simulink model "LQG"  (R2018b)
settings: Solver=FixedStepDiscrete  StartTime=0.0  StopTime=10  FixedStep=0.02  RelTol=1e-3  EnableMultiTasking=on
values from neighbouring files (symbols this model uses):
  A = [3.3545 -4.3521 2.6058 -0.6082; 1 0 0 0; 0 1 0 0; 0 0 1 0]    [LQGm.m]    (also in Testes_planta.m = [3.11506910744011 -3.74010634305672 2.06382118501694 -0.4387)
  B = [1;0;0;0]    [LQGm.m]    (also in Testes_planta.m)
  C = [-0.0657 0.1152 0 0]    [LQGm.m]    (also in Testes_planta.m = [-0.0767099115028891 0.161398714293952 0 0])
  Nbar = Nu+K*Nx    [LQGm.m]    (also in Testes_planta.m)
undefined symbols (not defined in the file or in its folder): K, M
settings Model: Creator=user  LastModifiedBy=joaj
settings DataIOCC: LimitDataPoints=on  SaveFormat=Array
settings OptimizationCC: LifeSpan=inf
settings DebuggingCC: SFUnexpectedBacktrackingDiag=warning  SFNoUnconditionalDefaultTransitionDiag=warning  SFExecutionAtInitializationDiag=none
settings HardwareCC: ProdBitPerPointer=32  ProdBitPerSizeT=32  ProdBitPerPtrDiffT=32  ProdLargestAtomicFloat=None  ProdIntDivRoundTo=Undefined  ProdEndianess=Unspecified  ProdWordSize=32  ProdHWDeviceType=32-bit Generic
settings ModelReferenceCC: PropagateSignalLabelsOutOfModel=off
settings SFSimCC: SimUseLocalCustomCode=off
settings RTWCC: RTWUseLocalCustomCode=off
settings CodeAppCC: StateflowObjectComments=on
settings GRTTargetCC: TargetLangStandard=C89/C90 (ANSI)  GeneratePreprocessorConditionals=Disable all
settings ConfigComp: CovMetricSettings=dw  CovHtmlReporting=on  CovSaveCumulativeToWorkspaceVar=on  CovSaveSingleToWorkspaceVar=on  CovExternalEMLEnable=off

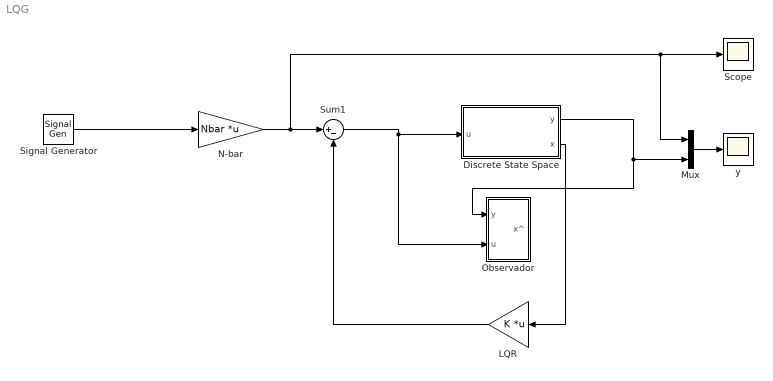
== system LQG ==
  "Discrete State Space " : Subsystem
  LQR : Gain  Gain=K  Multiplication=Matrix(K*u)
  Mux : Mux  Inputs=2
  N-bar : Gain  Gain=Nbar  Multiplication=Matrix(K*u)
  Observador : Subsystem
  Scope : Scope
  Signal Generator : SignalGenerator  WaveForm=square  Amplitude=90  Frequency=0.4
  Sum1 : Sum  Inputs=|+-
  y : Scope
  wires:
  LQR/1 -> Sum1/2
  "Discrete State Space "/1(y) -> Mux/2, Observador/1(y)
  Sum1/1 -> Observador/2(u), "Discrete State Space "/1(u)
  N-bar/1 -> Mux/1, Scope/1, Sum1/1
  "Discrete State Space "/2(x) -> LQR/1
  Signal Generator/1 -> N-bar/1
  Mux/1 -> y/1

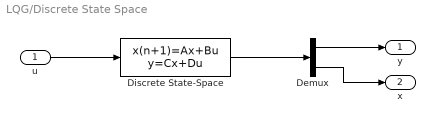
== system LQG/Discrete State Space  ==
  u : Inport
  Demux : Demux  Outputs=[1 length(A)]
  Discrete State-Space : DiscreteStateSpace  A=A  B=B  C=[C;eye(4)]  D=[0;0;0;0;0]  SampleTime=0.02
  y : Outport
  x : Outport  Port=2
  wires:
  Discrete State-Space/1 -> Demux/1
  Demux/1 -> y/1
  Demux/2 -> x/1
  u/1 -> Discrete State-Space/1

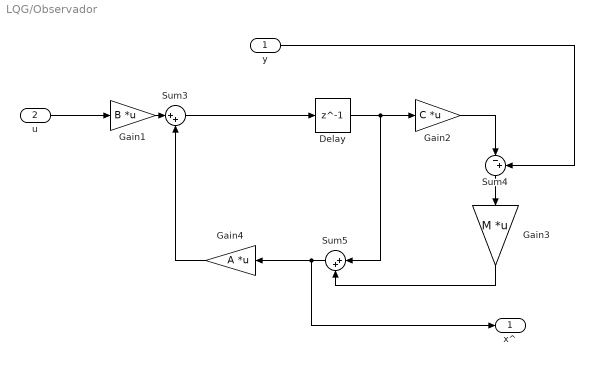
== system LQG/Observador ==
  y : Inport
  u : Inport  Port=2
  Delay : Delay  DelayLength=1  InitialCondition=0
  Gain1 : Gain  Gain=B  Multiplication=Matrix(K*u)
  Gain2 : Gain  Gain=C  Multiplication=Matrix(K*u)
  Gain3 : Gain  Gain=M  Multiplication=Matrix(K*u)
  Gain4 : Gain  Gain=A  Multiplication=Matrix(K*u)
  Sum3 : Sum  Inputs=|++
  Sum4 : Sum  Inputs=|-+
  Sum5 : Sum  Inputs=|++
  x^ : Outport
  wires:
  u/1 -> Gain1/1
  Gain1/1 -> Sum3/1
  Sum4/1 -> Gain3/1
  Gain3/1 -> Sum5/2
  Gain4/1 -> Sum3/2
  Sum5/1 -> x^/1, Gain4/1
  Delay/1 -> Sum5/1, Gain2/1
  Gain2/1 -> Sum4/1
  Sum3/1 -> Delay/1
  y/1 -> Sum4/2
